simulink model "task6"  (R2024a)
settings: Solver=VariableStepAuto  StartTime=0.0  StopTime=10.0  MaxStep=0.001  RelTol=1e-3
undefined symbols (not defined in the file): A, Abar, B, Bbar, Bfbar, C, D, Df, e0_bar, Gamma_w, Kw, Kx, L, w0, x0_hat, Yfbar, Ygbar
settings Model: Creator=sizgr  LastModifiedBy=sizgr

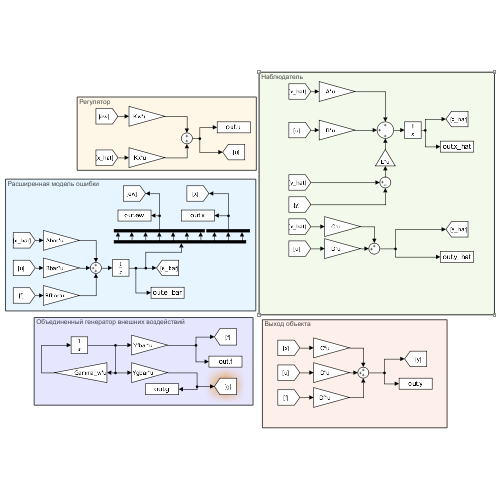
[thumbnail: Simulink's stored preview of the top-level diagram]
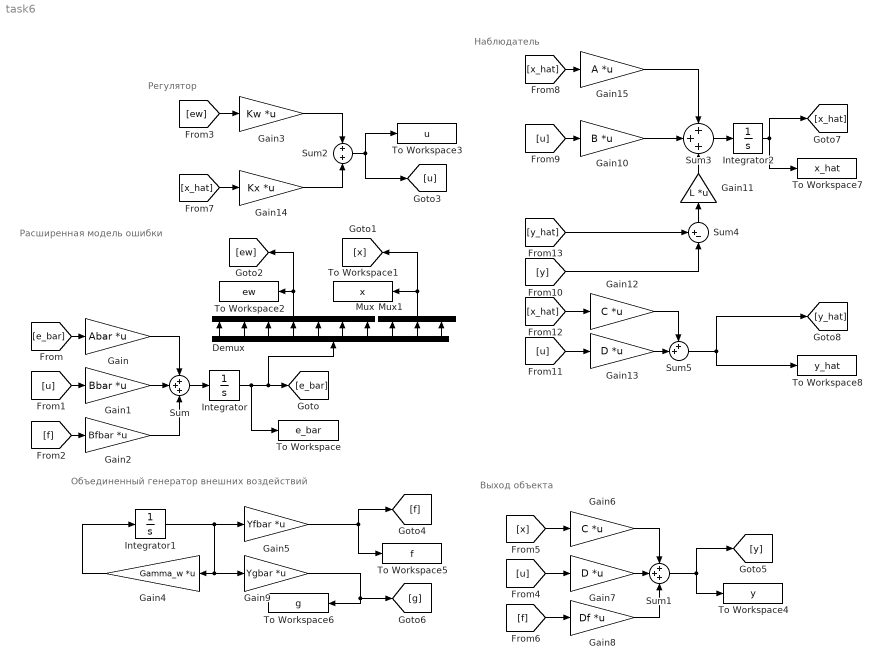
== system task6 ==
  note: Выход объекта
  note: Объединенный генератор внешних воздействий
  note: Расширенная модель ошибки
  note: Наблюдатель
  note: Регулятор
  Demux : Demux  Outputs=10
  Gain : Gain  Gain=Abar  Multiplication=Matrix(K*u)
  Gain1 : Gain  Gain=Bbar  Multiplication=Matrix(K*u)
  Gain10 : Gain  Gain=B  Multiplication=Matrix(K*u)
  Gain11 : Gain  Gain=L  Multiplication=Matrix(K*u)
  Gain12 : Gain  Gain=C  Multiplication=Matrix(K*u)
  Gain13 : Gain  Gain=D  Multiplication=Matrix(K*u)
  Gain14 : Gain  Gain=Kx  Multiplication=Matrix(K*u)
  Gain15 : Gain  Gain=A  Multiplication=Matrix(K*u)
  Gain2 : Gain  Gain=Bfbar  Multiplication=Matrix(K*u)
  Gain3 : Gain  Gain=Kw  Multiplication=Matrix(K*u)
  Gain4 : Gain  Gain=Gamma_w  Multiplication=Matrix(K*u)
  Gain5 : Gain  Gain=Yfbar  Multiplication=Matrix(K*u)
  Gain6 : Gain  Gain=C  Multiplication=Matrix(K*u)
  Gain7 : Gain  Gain=D  Multiplication=Matrix(K*u)
  Gain8 : Gain  Gain=Df  Multiplication=Matrix(K*u)
  Gain9 : Gain  Gain=Ygbar  Multiplication=Matrix(K*u)
  Integrator : Integrator  InitialCondition=e0_bar
  Integrator1 : Integrator  InitialCondition=w0
  Integrator2 : Integrator  InitialCondition=x0_hat
  Mux : Mux  Inputs=7
  Mux1 : Mux  Inputs=3
  Sum : Sum  Inputs=+++
  Sum1 : Sum  Inputs=+++
  Sum2 : Sum  Inputs=+|+
  Sum3 : Sum  Inputs=+++
  Sum4 : Sum  Inputs=+-|
  Sum5 : Sum  Inputs=++|
  To Workspace : ToWorkspace  VariableName=e_bar  SaveFormat=Timeseries  SampleTime=-1
  To Workspace1 : ToWorkspace  VariableName=x  SaveFormat=Timeseries  SampleTime=-1
  To Workspace2 : ToWorkspace  VariableName=ew  SaveFormat=Timeseries  SampleTime=-1
  To Workspace3 : ToWorkspace  VariableName=u  SaveFormat=Timeseries  SampleTime=-1
  To Workspace4 : ToWorkspace  VariableName=y  SaveFormat=Timeseries  SampleTime=-1
  To Workspace5 : ToWorkspace  VariableName=f  SaveFormat=Timeseries  SampleTime=-1
  To Workspace6 : ToWorkspace  VariableName=g  SaveFormat=Timeseries  SampleTime=-1
  To Workspace7 : ToWorkspace  VariableName=x_hat  SaveFormat=Timeseries  SampleTime=-1
  To Workspace8 : ToWorkspace  VariableName=y_hat  SaveFormat=Timeseries  SampleTime=-1
  wires:
  Sum/1 -> Integrator/1
  Integrator/1 -> Demux/1, [e_bar], To Workspace/1
  [e_bar] -> Gain/1
  [u] -> Gain1/1
  [f] -> Gain2/1
  Gain1/1 -> Sum/2
  Gain/1 -> Sum/1
  Gain2/1 -> Sum/3
  Integrator1/1 -> Gain5/1, Gain9/1, Gain4/1
  Gain4/1 -> Integrator1/1
  Gain5/1 -> [f], To Workspace5/1
  Gain6/1 -> Sum1/1
  Gain7/1 -> Sum1/2
  [u] -> Gain7/1
  [x] -> Gain6/1
  Sum1/1 -> To Workspace4/1, [y]
  [f] -> Gain8/1
  Gain8/1 -> Sum1/3
  Demux/1 -> Mux/1
  Demux/2 -> Mux/2
  Demux/3 -> Mux/3
  Mux/1 -> [ew], To Workspace2/1
  Mux1/1 -> [x], To Workspace1/1
  Demux/4 -> Mux/4
  Gain9/1 -> To Workspace6/1, [g]
  Demux/5 -> Mux/5
  Demux/6 -> Mux/6
  Demux/7 -> Mux/7
  Demux/8 -> Mux1/1
  Demux/9 -> Mux1/2
  Demux/10 -> Mux1/3
  Integrator2/1 -> To Workspace7/1, [x_hat]
  [x_hat] -> Gain15/1
  [u] -> Gain13/1
  [ew] -> Gain3/1
  Gain13/1 -> Sum5/2
  [u] -> Gain10/1
  Sum5/1 -> To Workspace8/1, [y_hat]
  Gain14/1 -> Sum2/2
  Sum3/1 -> Integrator2/1
  [x_hat] -> Gain12/1
  [y_hat] -> Sum4/1
  Gain15/1 -> Sum3/1
  [x_hat] -> Gain14/1
  Gain12/1 -> Sum5/1
  Sum2/1 -> To Workspace3/1, [u]
  [y] -> Sum4/2
  Gain3/1 -> Sum2/1
  Gain10/1 -> Sum3/2
  Gain11/1 -> Sum3/3
  Sum4/1 -> Gain11/1
